simulink model "BuckThreePhaseTEST7_PID_2_8"  (R2013b)
settings: Solver=ode45  StartTime=0.0  StopTime=0.01  MaxStep=1e-6  RelTol=1e-3
libraries: powerlib x19, simulink x5, simulink_need_slupdate x1
settings Model: Creator=Cristi  LastModifiedBy=Cristi
settings DebuggingCC: MaxConsecutiveZCsMsg=none

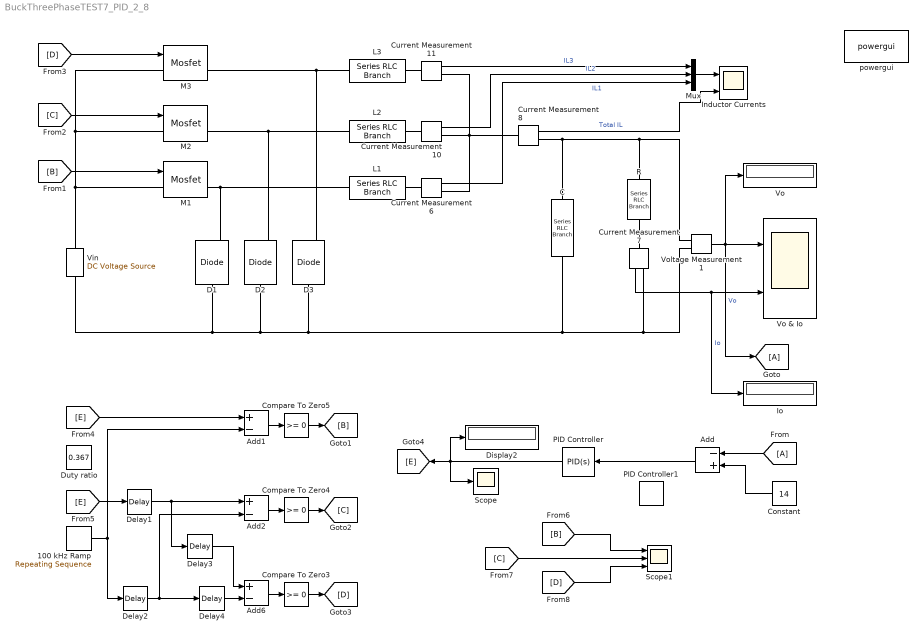
== system BuckThreePhaseTEST7_PID_2_8 ==
  " C " : powerlib/Elements/Series RLC Branch  LConnTagsString=__new0  RConnTagsString=__new0  BranchType=C  Resistance=0.01  Inductance=1e-3  SetiL0=off  InitialCurrent=0  Capacitance=300e-6  Setx0=off  InitialVoltage=0  Measurements=None
  100 kHz Ramp : simulink/Sources/Repeating Sequence  rep_seq_t=[0 1/100000]  rep_seq_y=[0 1]
  Add : Sum  Inputs=-+
  Add1 : Sum  Inputs=+-
  Add2 : Sum  Inputs=+-
  Add6 : Sum  Inputs=+-
  Compare To Zero3 : simulink/Logic and Bit Operations/Compare To Zero  relop=>=  OutDataTypeStr=uint8
  Compare To Zero4 : simulink/Logic and Bit Operations/Compare To Zero  relop=>=  OutDataTypeStr=uint8
  Compare To Zero5 : simulink/Logic and Bit Operations/Compare To Zero  relop=>=  OutDataTypeStr=uint8
  Constant : Constant  Value=14
  Current Measurement{6..8,10..11} (5 alike) : powerlib/Measurements/Current Measurement  PhasorSimulation=off  OutputType=Complex  PSBequivalent=0
  D1 : powerlib/Power Electronics/Diode  Ron=0.001  Lon=0  Vf=0.7  IC=0  UseSnubber=off  Rs=500  Cs=250e-9  Measurements=on
  D2 : powerlib/Power Electronics/Diode  Ron=0.001  Lon=0  Vf=0.7  IC=0  UseSnubber=off  Rs=500  Cs=250e-9  Measurements=on
  D3 : powerlib/Power Electronics/Diode  Ron=0.001  Lon=0  Vf=0.7  IC=0  UseSnubber=off  Rs=500  Cs=250e-9  Measurements=on
  Delay1 : TransportDelay  DelayTime=3.3333e-06
  Delay2 : TransportDelay  DelayTime=3.3333e-06
  "Delay3 " : TransportDelay  DelayTime=3.3333e-06
  Delay4 : TransportDelay  DelayTime=3.3333e-06
  Display2 : Display
  Duty ratio : Constant  Value=0.367
  Inductor Currents : Scope  NumInputPorts=2
      settings: TimeRange=7.919136237782235e-05  YMin=0.9330985915492818~0  YMax=47.83450704225351~180
  Io : Display
  L1 : powerlib/Elements/Series RLC Branch  LConnTagsString=__new0  RConnTagsString=__new0  BranchType=L  Resistance=1  Inductance=2.8e-4  SetiL0=off  InitialCurrent=0  Capacitance=1e-6  Setx0=off  InitialVoltage=0  Measurements=None
  L2 : powerlib/Elements/Series RLC Branch  LConnTagsString=__new0  RConnTagsString=__new0  BranchType=L  Resistance=1  Inductance=2.8e-4  SetiL0=off  InitialCurrent=0  Capacitance=1e-6  Setx0=off  InitialVoltage=0  Measurements=None
  L3 : powerlib/Elements/Series RLC Branch  LConnTagsString=__new0  RConnTagsString=__new0  BranchType=L  Resistance=1  Inductance=2.8e-4  SetiL0=off  InitialCurrent=0  Capacitance=1e-6  Setx0=off  InitialVoltage=0  Measurements=None
  M1 : powerlib/Power Electronics/Mosfet  Ron=0.1  Lon=0  Rd=0.01  Vfd=0  IC=0  Rs=1e5  Cs=inf  Measurements=on
  M2 : powerlib/Power Electronics/Mosfet  Ron=0.1  Lon=0  Rd=0.01  Vfd=0  IC=0  Rs=1e5  Cs=inf  Measurements=on
  M3 : powerlib/Power Electronics/Mosfet  Ron=0.1  Lon=0  Rd=0.01  Vfd=0  IC=0  Rs=1e5  Cs=inf  Measurements=on
  Mux : Mux  Inputs=3
  PID Controller : simulink/Continuous/PID Controller  Controller=PID  TimeDomain=Continuous-time  SampleTime=1  IntegratorMethod=Forward Euler  FilterMethod=Forward Euler  Form=Parallel  P=0.04  I=240  D=0.00001  N=100  InitialConditionSource=internal  InitialConditionForIntegrator=0  InitialConditionForFilter=0  ExternalReset=none  LimitOutput=off  UpperSaturationLimit=inf  LowerSaturationLimit=-inf  LinearizeAsGain=on  AntiWindupMode=none  Kb=1  TrackingMode=off  Kt=1  PParamMin=[]  PParamMax=[]  IParamMin=[]  IParamMax=[]  DParamMin=[]  DParamMax=[]  NParamMin=[]  NParamMax=[]  KbParamMin=[]  KbParamMax=[]  KtParamMin=[]  KtParamMax=[]  POutMin=[]  POutMax=[]  IOutMin=[]  IOutMax=[]  DOutMin=[]  DOutMax=[]  NOutMin=[]  NOutMax=[]  KbOutMin=[]  KbOutMax=[]  KtOutMin=[]  KtOutMax=[]  IntegratorOutMin=[]  IntegratorOutMax=[]  FilterOutMin=[]  FilterOutMax=[]  SumOutMin=[]  SumOutMax=[]  SumI1OutMin=[]  SumI1OutMax=[]  SumI2OutMin=[]  SumI2OutMax=[]  SumI3OutMin=[]  SumI3OutMax=[]  SumDOutMin=[]  SumDOutMax=[]  SaturationOutMin=[]  SaturationOutMax=[]  IntegratorContinuousStateAttributes=''  IntegratorStateMustResolveToSignalObject=off  IntegratorRTWStateStorageClass=Auto  FilterContinuousStateAttributes=''  FilterStateMustResolveToSignalObject=off  FilterRTWStateStorageClass=Auto
  PID Controller1 : simulink_need_slupdate/PID Controller  P=5  I=1  D=0
  R : powerlib/Elements/Series RLC Branch  LConnTagsString=__new0  RConnTagsString=__new0  BranchType=R  Resistance=0.197  Inductance=1e-3  SetiL0=off  InitialCurrent=0  Capacitance=1e-6  Setx0=off  InitialVoltage=0  Measurements=None
  Scope : Scope
      settings: SaveName=ScopeData2
  Scope1 : Scope  NumInputPorts=3
      settings: TimeRange=0.0002395510286625671  YMin=-0.5~-2~-2  YMax=1.5~2~2  SaveName=ScopeData3
  Vin : powerlib/Electrical Sources/DC Voltage Source  Amplitude=42  Measurements=None
  Vo : Display
  Vo & Io : Scope  NumInputPorts=2
      settings: YMin=11.1~56.4  YMax=11.4~57.8
  Voltage Measurement1 : powerlib/Measurements/Voltage Measurement  PhasorSimulation=off  OutputType=Complex  PSBequivalent=0
  powergui : powerlib/powergui  Priority=1  SimulationMode=Continuous  SolverType=Tustin  SampleTime=50e-6  frequency=60  SPID=off  DisableSnubberDevices=off  DisableRonSwitches=off  DisableVfSwitches=off  SwTol=0  Interpol=off  DisplayEquations=off  frequencyindice=0  Pbase=100e6  ErrMax=1e-4  Iterations=50  UnitsV=kV  UnitsW=MW  FunctionMessages=off  echomessages=off  HookPort=off  EnableUseOfTLC=off  x0status=steady  RestoreLinks=warning  ResistiveCurrentMeasurement=off  Frange=[0:2:500]  Ylog=off  Xlog=on  ShowGrid=off  save=off  variable=ZData  ZoomFFT=off  StartTime=0.0  cycles=1  DisplayStyle=1  fundamental=60  FreqAxis=off  MaxFrequency=1000  frequencyindicesteady=1  RmsSteady=1  display=off  Ts=0  methode=off
  wires:
  Delay1/1 -> Add2/1, "Delay3 "/1
  Delay2/1 -> Delay4/1, Add2/2
  "Delay3 "/1 -> Add6/1
  Delay4/1 -> Add6/2
  Add6/1 -> Compare To Zero3/1
  Add2/1 -> Compare To Zero4/1
  Add1/1 -> Compare To Zero5/1
  Voltage Measurement1/1 -> [A], Vo/1, Vo & Io/1  "Vo"
  Current Measurement7/1 -> Io/1, Vo & Io/2  "Io"
  Current Measurement11/1 -> Mux/1  "IL3"
  Current Measurement10/1 -> Mux/2  "IL2"
  Mux/1 -> Inductor Currents/1
  Current Measurement6/1 -> Mux/3  "IL1"
  Current Measurement8/1 -> Inductor Currents/2  "Total IL"
  100 kHz Ramp/1 -> Delay2/1, Add1/2
  Constant/1 -> Add/2
  [A] -> Add/1
  PID Controller/1 -> [E], Scope/1, Display2/1
  Add/1 -> PID Controller/1
  Compare To Zero5/1 -> [B]
  [B] -> M1/1
  Compare To Zero4/1 -> [C]
  [C] -> M2/1
  Compare To Zero3/1 -> [D]
  [D] -> M3/1
  [E] -> Add1/1
  [E] -> Delay1/1
  [B] -> Scope1/1
  [C] -> Scope1/2
  [D] -> Scope1/3
  connections:
  L1/LConn1 -- D1/RConn1 -- M1/RConn1
  D2/RConn1 -- L2/LConn1 -- M2/RConn1
  L3/LConn1 -- M3/RConn1 -- D3/RConn1
  Current Measurement6/RConn1 -- Current Measurement10/RConn1 -- Current Measurement8/LConn1 -- Current Measurement11/RConn1
  Vin/LConn1 -- D3/LConn1 -- " C "/RConn1 -- Voltage Measurement1/LConn2 -- Current Measurement7/RConn1 -- D2/LConn1 -- D1/LConn1
  Voltage Measurement1/LConn1 -- R/LConn1 -- " C "/LConn1 -- Current Measurement8/RConn1
  M3/LConn1 -- Vin/RConn1 -- M1/LConn1 -- M2/LConn1
  Current Measurement7/LConn1 -- R/RConn1
  Current Measurement11/LConn1 -- L3/RConn1
  L2/RConn1 -- Current Measurement10/LConn1
  Current Measurement6/LConn1 -- L1/RConn1
